simulink model "msk_syn_cordic"  (Simulink 7.9)
settings: Solver=FixedStepDiscrete  SolverMode=SingleTasking  StartTime=0.0  StopTime=100  RelTol=1e-3
PreLoadFcn:
  | msk_syn_init;
undefined symbols (not defined in the file or in its folder): msk_syn_params
libraries: shlslibv1 x10
settings Model: synDspstartup=OK  Creator=sszilvasi  LastModifiedBy=sszilvasi
settings DataIOCC: SaveOutput=off  SignalLogging=off  SaveTime=off
settings OptimizationCC: InlineParams=on
settings DebuggingCC: AlgebraicLoopMsg=error

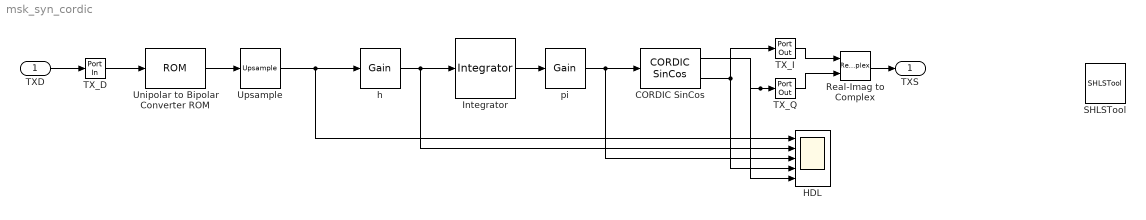
== system msk_syn_cordic ==
  TXD : Inport
  CORDIC SinCos : shlslibv1/CORDIC/CORDIC SinCos  syn_sincos_opr=sin&cos  syn_iter_nb=10  syn_out_wl=10  synBlockType=primitive  synLatency=12  synBlockId=53
  HDL : Scope  NumInputPorts=5
      settings: YMin=-5~-5~-5~-5~-5  YMax=5~5~5~5~5
  Integrator : shlslibv1/Filtering/Integrator  syn_pole_val=1  syn_feedback_fl=8  syn_out_f=Automatic  syn_out_wl=16  syn_out_fl=8  syn_out_dt=signed  syn_out_sat=off  syn_out_rnd=off  syn_rst_port=off  syn_en_port=off  synBlockType=custom  synLatency=0
  Real-Imag to Complex : RealImagToComplex
  SHLSTool : shlslibv1/SHLSTool  synBlockType=tool  syn_dsp_mode=FPGA
  TX_D : shlslibv1/Ports & Subsystems/Port In  syn_out_wl=1  syn_out_fl=0  syn_out_dt=unsigned  syn_out_st=1  syn_capture=off  syn_register=off  syn_out_sat=off  syn_out_rnd=on  synBlockType=port  synLatency=0  synBlockId=0
  TX_I : shlslibv1/Ports & Subsystems/Port Out  syn_capture=off  syn_register=off  synBlockType=port  synLatency=0  synBlockId=1
  TX_Q : shlslibv1/Ports & Subsystems/Port Out  syn_capture=off  syn_register=off  synBlockType=port  synLatency=0  synBlockId=1
  Unipolar to Bipolar Converter ROM : shlslibv1/Memories/ROM  syn_rom_vec=[-1 1]  syn_out_wl=16  syn_out_fl=14  syn_out_dt=signed  syn_out_sat=off  syn_out_rnd=on  synBlockType=primitive  synLatency=1  synBlockId=62
  Upsample : shlslibv1/Signal Operations/Upsample  syn_r_val=msk_syn_params.N  syn_in_hold=on  syn_sample_offset=0  syn_sync_mode=No Sync  synBlockType=primitive  synLatency=0  synBlockId=6
  h : shlslibv1/Math Functions/Gain  syn_gain_val=1/2*1/msk_syn_params.N  syn_gain_fl=15  syn_gain_dt=signed  syn_gain_rnd=on  syn_out_f=Full Precision  syn_out_wl=16  syn_out_fl=8  syn_out_dt=signed  syn_out_sat=off  syn_out_rnd=Floor (Truncate)  synBlockType=primitive  synLatency=0  synBlockId=3  syn_opr_mode=0
  pi : shlslibv1/Math Functions/Gain  syn_gain_val=1/2  syn_gain_fl=15  syn_gain_dt=signed  syn_gain_rnd=on  syn_out_f=Full Precision  syn_out_wl=16  syn_out_fl=8  syn_out_dt=signed  syn_out_sat=off  syn_out_rnd=Floor (Truncate)  synBlockType=primitive  synLatency=0  synBlockId=3  syn_opr_mode=0
  TXS : Outport
  wires:
  Upsample/1 -> HDL/1, h/1
  TX_D/1 -> Unipolar to Bipolar Converter ROM/1
  Unipolar to Bipolar Converter ROM/1 -> Upsample/1
  TX_I/1 -> Real-Imag to Complex/1
  TX_Q/1 -> Real-Imag to Complex/2
  h/1 -> HDL/2, Integrator/1
  Integrator/1 -> pi/1
  pi/1 -> CORDIC SinCos/1, HDL/3
  CORDIC SinCos/2 -> TX_I/1, HDL/4
  CORDIC SinCos/1 -> HDL/5, TX_Q/1
  TXD/1 -> TX_D/1
  Real-Imag to Complex/1 -> TXS/1
